simulink library "SEMACE2_IN"  (R2021b)
settings: Solver=VariableStepAuto  StartTime=0.0  StopTime=10.0  RelTol=1e-3
values from neighbouring files (symbols this model uses):
  dataSEMACE = 60.0    [applicationDD.sldd]    (also in dataSEMACE.mat = ; dataSEMACE_DD.sldd)
settings Model: Creator=ACH  LastModifiedBy=ACH

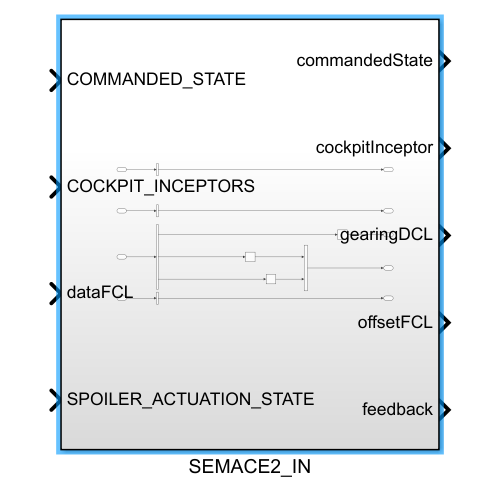
[thumbnail: Simulink's stored preview of the top-level diagram]
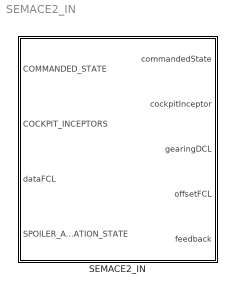
== system SEMACE2_IN ==
  SEMACE2_IN : Subsystem

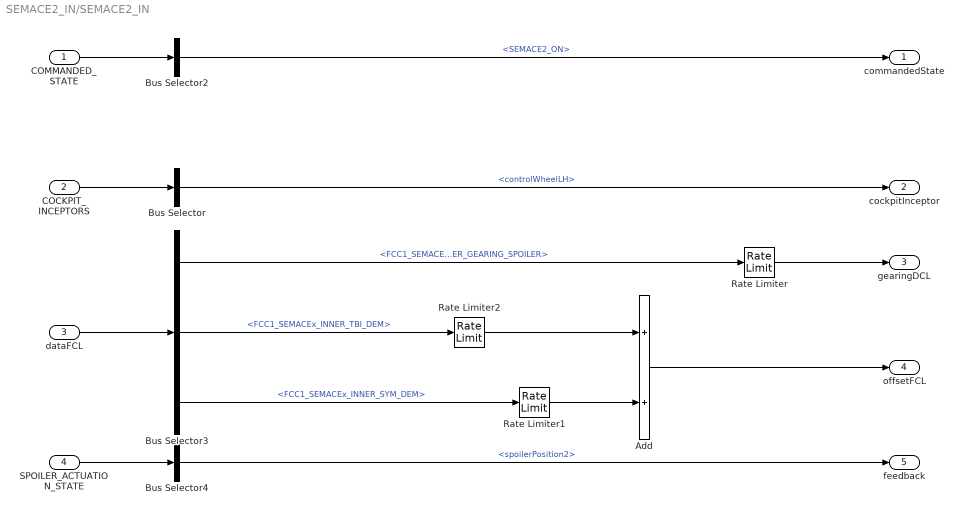
== system SEMACE2_IN/SEMACE2_IN ==
  COMMANDED_STATE : Inport  OutDataTypeStr=Bus: COMMANDED_STATE
  COCKPIT_INCEPTORS : Inport  Port=2  OutDataTypeStr=Bus: COCKPIT_INCEPTORS
  dataFCL : Inport  Port=3  OutDataTypeStr=Bus: FCC1_SEMACEx_INNER_C1
  SPOILER_ACTUATION_STATE : Inport  Port=4  OutDataTypeStr=Bus: SPOILER_ACTUATION_STATE
  Add : Sum
  Bus Selector : BusSelector  OutputSignals=controlWheelLH
  Bus Selector2 : BusSelector  OutputSignals=SEMACE2_ON
  Bus Selector3 : BusSelector  OutputSignals=FCC1_SEMACEx_INNER_GEARING_SPOILER,FCC1_SEMACEx_INNER_TBI_DEM,FCC1_SEMACEx_INNER_SYM_DEM
  Bus Selector4 : BusSelector  OutputSignals=spoilerPosition2
  Rate Limiter : RateLimiter  RisingSlewLimit=dataSEMACE.rateLimiterGearing  FallingSlewLimit=-dataSEMACE.rateLimiterGearing  SampleTimeMode=inherited
      settings: AttributesFormatString=|
      | %<RisingSlewLimit>
      | %<FallingSlewLimit>
  Rate Limiter1 : RateLimiter  RisingSlewLimit=dataSEMACE.rateLimiterSymmetric  FallingSlewLimit=-dataSEMACE.rateLimiterSymmetric  SampleTimeMode=inherited
      settings: AttributesFormatString=|
      | %<RisingSlewLimit>
      | %<FallingSlewLimit>
  Rate Limiter2 : RateLimiter  RisingSlewLimit=dataSEMACE.rateLimiterTBI  FallingSlewLimit=-dataSEMACE.rateLimiterTBI  SampleTimeMode=inherited
      settings: AttributesFormatString=|
      | %<RisingSlewLimit>
      | %<FallingSlewLimit>
  commandedState : Outport
  cockpitInceptor : Outport  Port=2
  gearingDCL : Outport  Port=3
  offsetFCL : Outport  Port=4
  feedback : Outport  Port=5
  wires:
  Bus Selector3/2 -> Rate Limiter2/1  "<FCC1_SEMACEx_INNER_TBI_DEM>"
  Add/1 -> offsetFCL/1
  Bus Selector3/3 -> Rate Limiter1/1  "<FCC1_SEMACEx_INNER_SYM_DEM>"
  SPOILER_ACTUATION_STATE/1 -> Bus Selector4/1
  Bus Selector2/1 -> commandedState/1  "<SEMACE2_ON>"
  Bus Selector4/1 -> feedback/1  "<spoilerPosition2>"
  COMMANDED_STATE/1 -> Bus Selector2/1
  dataFCL/1 -> Bus Selector3/1
  COCKPIT_INCEPTORS/1 -> Bus Selector/1
  Bus Selector/1 -> cockpitInceptor/1  "<controlWheelLH>"
  Bus Selector3/1 -> Rate Limiter/1  "<FCC1_SEMACEx_INNER_GEARING_SPOILER>"
  Rate Limiter1/1 -> Add/2
  Rate Limiter/1 -> gearingDCL/1
  Rate Limiter2/1 -> Add/1
